simulink model "nolineal_closeloop_referencia_yr"  (R2014a)
settings: Solver=ode15s  StartTime=0.0  StopTime=900  RelTol=1e-3
libraries: simulink x2
settings Model: Creator=JuanPablo  LastModifiedBy=juanr
settings DataIOCC: SignalLoggingSaveFormat=ModelDataLogs
settings OptimizationCC: ExpressionDepthLimit=2147483647
settings DebuggingCC: AlgebraicLoopMsg=none  UnderspecifiedInitializationDetection=Classic  FcnCallInpInsideContextMsg=EnableAllAsWarning  StateNameClashWarn=warning

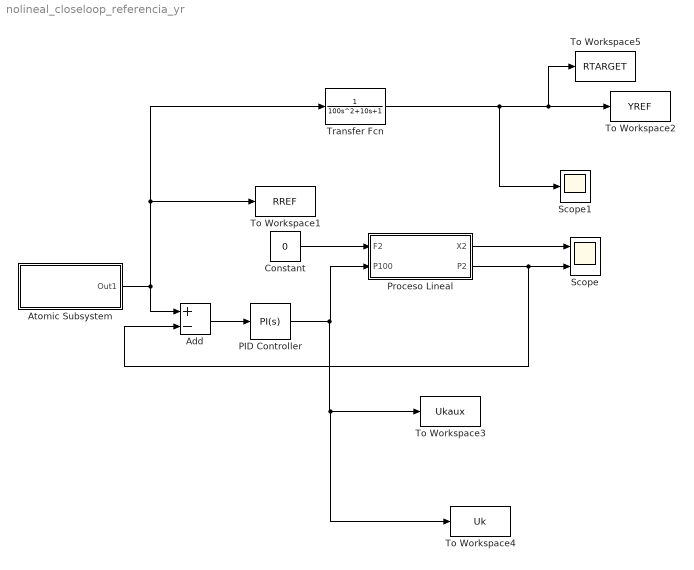
== system nolineal_closeloop_referencia_yr ==
  Add : Sum  Inputs=+-
  Atomic Subsystem : Subsystem  TreatAsAtomicUnit=on
  Constant : Constant  Value=0
  PID Controller : simulink/Continuous/PID Controller  Controller=PI  TimeDomain=Continuous-time  SampleTime=1  IntegratorMethod=Forward Euler  FilterMethod=Forward Euler  Form=Parallel  P=2.3284  I=2.3284/9.8648  D=0  N=100  InitialConditionSource=internal  InitialConditionForIntegrator=0  InitialConditionForFilter=0  ExternalReset=none  LimitOutput=off  UpperSaturationLimit=inf  LowerSaturationLimit=-inf  LinearizeAsGain=on  AntiWindupMode=none  Kb=1  TrackingMode=off  Kt=1  PParamMin=[]  PParamMax=[]  IParamMin=[]  IParamMax=[]  DParamMin=[]  DParamMax=[]  NParamMin=[]  NParamMax=[]  KbParamMin=[]  KbParamMax=[]  KtParamMin=[]  KtParamMax=[]  POutMin=[]  POutMax=[]  IOutMin=[]  IOutMax=[]  DOutMin=[]  DOutMax=[]  NOutMin=[]  NOutMax=[]  KbOutMin=[]  KbOutMax=[]  KtOutMin=[]  KtOutMax=[]  IntegratorOutMin=[]  IntegratorOutMax=[]  FilterOutMin=[]  FilterOutMax=[]  SumOutMin=[]  SumOutMax=[]  SumI1OutMin=[]  SumI1OutMax=[]  SumI2OutMin=[]  SumI2OutMax=[]  SumI3OutMin=[]  SumI3OutMax=[]  SumDOutMin=[]  SumDOutMax=[]  SaturationOutMin=[]  SaturationOutMax=[]  IntegratorContinuousStateAttributes=''  IntegratorStateMustResolveToSignalObject=off  IntegratorRTWStateStorageClass=Auto  FilterContinuousStateAttributes=''  FilterStateMustResolveToSignalObject=off  FilterRTWStateStorageClass=Auto
  Proceso Lineal : Subsystem  TreatAsAtomicUnit=on
  Scope : Scope  NumInputPorts=2
      settings: TimeRange=400  YMin=-1~0  YMax=1~0.14  SaveName=openloop
  Scope1 : Scope
  To Workspace1 : ToWorkspace  VariableName=RREF  SaveFormat=Timeseries  SampleTime=5
  To Workspace2 : ToWorkspace  VariableName=YREF  SaveFormat=Timeseries  SampleTime=5
  To Workspace3 : ToWorkspace  VariableName=Ukaux  SaveFormat=Timeseries  SampleTime=5
  To Workspace4 : ToWorkspace  VariableName=Uk  SaveFormat=Timeseries  SampleTime=5
  To Workspace5 : ToWorkspace  VariableName=RTARGET  SaveFormat=Timeseries  SampleTime=5
  Transfer Fcn : TransferFcn  Denominator=[100 10 1]
  wires:
  Proceso Lineal/1(X2) -> Scope/1
  Constant/1 -> Proceso Lineal/1("F2 ")
  Add/1 -> PID Controller/1
  Atomic Subsystem/1(Out1) -> Transfer Fcn/1, To Workspace1/1, Add/1
  Proceso Lineal/2(P2) -> Add/2, Scope/2
  PID Controller/1 -> Proceso Lineal/2(P100), To Workspace4/1, To Workspace3/1
  Transfer Fcn/1 -> Scope1/1, To Workspace5/1, To Workspace2/1

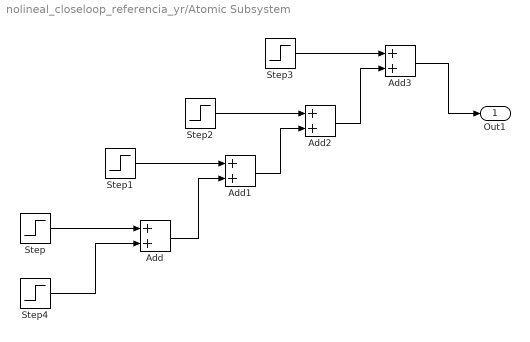
== system nolineal_closeloop_referencia_yr/Atomic Subsystem ==
  Add{,1..3} (4 alike) : Sum
  Step : Step  Time=300  After=0.05  SampleTime=0
  Step1 : Step  Time=600  After=0.05  SampleTime=0
  Step2 : Step  Time=450  After=0  SampleTime=0
  Step3 : Step  Time=200  After=0  SampleTime=0
  Step4 : Step  Time=0  Before=0.1  After=0.1  SampleTime=0
  Out1 : Outport
  wires:
  Step/1 -> Add/1
  Step1/1 -> Add1/1
  Add/1 -> Add1/2
  Step2/1 -> Add2/1
  Add1/1 -> Add2/2
  Step3/1 -> Add3/1
  Add2/1 -> Add3/2
  Add3/1 -> Out1/1
  Step4/1 -> Add/2

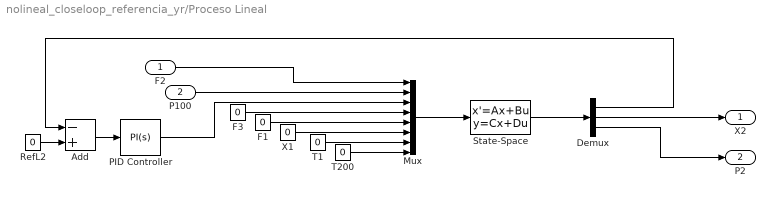
== system nolineal_closeloop_referencia_yr/Proceso Lineal ==
  "F2 " : Inport
  P100 : Inport  Port=2
  Add : Sum  Inputs=-+
  Demux : Demux  Outputs=3
  F1 : Constant  Value=0
  F3 : Constant  Value=0
  Mux : Mux  Inputs=8
  PID Controller : simulink/Continuous/PID Controller  Controller=PI  TimeDomain=Continuous-time  SampleTime=1  IntegratorMethod=Forward Euler  FilterMethod=Forward Euler  Form=Parallel  P=-0.601  I=-0.601/92.671  D=0  N=100  InitialConditionSource=internal  InitialConditionForIntegrator=0  InitialConditionForFilter=0  ExternalReset=none  LimitOutput=off  UpperSaturationLimit=inf  LowerSaturationLimit=-inf  LinearizeAsGain=on  AntiWindupMode=none  Kb=1  TrackingMode=off  Kt=1  PParamMin=[]  PParamMax=[]  IParamMin=[]  IParamMax=[]  DParamMin=[]  DParamMax=[]  NParamMin=[]  NParamMax=[]  KbParamMin=[]  KbParamMax=[]  KtParamMin=[]  KtParamMax=[]  POutMin=[]  POutMax=[]  IOutMin=[]  IOutMax=[]  DOutMin=[]  DOutMax=[]  NOutMin=[]  NOutMax=[]  KbOutMin=[]  KbOutMax=[]  KtOutMin=[]  KtOutMax=[]  IntegratorOutMin=[]  IntegratorOutMax=[]  FilterOutMin=[]  FilterOutMax=[]  SumOutMin=[]  SumOutMax=[]  SumI1OutMin=[]  SumI1OutMax=[]  SumI2OutMin=[]  SumI2OutMax=[]  SumI3OutMin=[]  SumI3OutMax=[]  SumDOutMin=[]  SumDOutMax=[]  SaturationOutMin=[]  SaturationOutMax=[]  IntegratorContinuousStateAttributes=''  IntegratorStateMustResolveToSignalObject=off  IntegratorRTWStateStorageClass=Auto  FilterContinuousStateAttributes=''  FilterStateMustResolveToSignalObject=off  FilterRTWStateStorageClass=Auto
  "RefL2 " : Constant  Value=0
  State-Space : StateSpace  A=[0 0.10455 0.37935; 0 -0.1 0; 0 -0.10340e-1 -0.54738e-1]  B=[-0.1 -0.37266 0 -0.36676 0.38605 0 -0.3636e-1 0; -0.1 0 0 0 0.1 0.1 0 0; 0 0.36914e-1 -0.75272e-2 0.36302e-1 0.32268e-2 0 0.35972e-2 0.17785e-1]  C=[1 0 0; 0 1 0; 0 0 1]  D=zeros(3,8)  X0=0
  T1 : Constant  Value=0
  T200 : Constant  Value=0
  X1 : Constant  Value=0
  X2 : Outport
  P2 : Outport  Port=2
  wires:
  Mux/1 -> State-Space/1
  State-Space/1 -> Demux/1
  "F2 "/1 -> Mux/1
  P100/1 -> Mux/2
  PID Controller/1 -> Mux/3
  F3/1 -> Mux/4
  F1/1 -> Mux/5
  X1/1 -> Mux/6
  T1/1 -> Mux/7
  T200/1 -> Mux/8
  Demux/1 -> Add/1
  Demux/2 -> X2/1
  Demux/3 -> P2/1
  Add/1 -> PID Controller/1
  "RefL2 "/1 -> Add/2
